simulink model "model_06"  (R2021b)
settings: Solver=VariableStepAuto  StartTime=0  StopTime=60  RelTol=1e-3
settings Model: Creator=jimd  LastModifiedBy=jimd

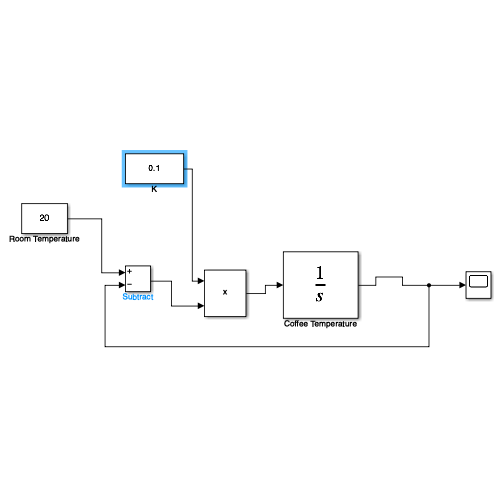
[thumbnail: Simulink's stored preview of the top-level diagram]
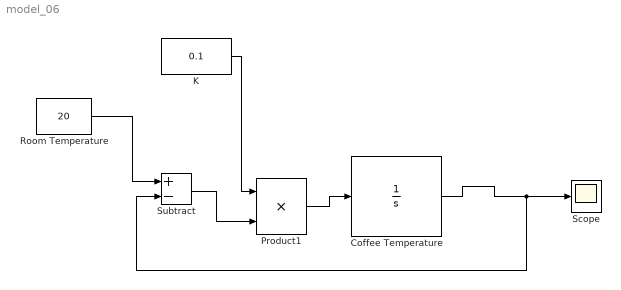
== system model_06 ==
  Coffee Temperature : Integrator  InitialCondition=80
  K : Constant  Value=0.1
  Product1 : Product
  Room Temperature : Constant  Value=20
  Scope : Scope
  Subtract : Sum  Inputs=+-
  wires:
  Coffee Temperature/1 -> Subtract/2, Scope/1
  Product1/1 -> Coffee Temperature/1
  Room Temperature/1 -> Subtract/1
  K/1 -> Product1/1
  Subtract/1 -> Product1/2
